simulink model "SF031A_CurrReasbnDiagc"  (R2013b)
settings: Solver=FixedStepDiscrete  SolverMode=SingleTasking  StartTime=0.0  StopTime=1  FixedStep=0.000125  RelTol=1e-3
values from neighbouring files (symbols this model uses):
  ARCHGLBPRM_2MILLISEC_SEC_F32 = DataDict.Constant    [SF031A_CurrReasbnDiagc_DataDict.m]
  ARCHGLBPRM_2PI_ULS_F32 = DataDict.Constant    [SF031A_CurrReasbnDiagc_DataDict.m]
  CurrReasbnDiagcCurrDiagcMotEnvlpTblMax = DataDict.Calibration    [SF031A_CurrReasbnDiagc_DataDict.m]
  CurrReasbnDiagcCurrDiagcPrimErrThd = DataDict.Calibration    [SF031A_CurrReasbnDiagc_DataDict.m]
  CurrReasbnDiagcCurrDiagcSecdryErrThd = DataDict.Calibration    [SF031A_CurrReasbnDiagc_DataDict.m]
  CurrReasbnDiagcCurrDiagcSecdryTqLimThd = DataDict.Calibration    [SF031A_CurrReasbnDiagc_DataDict.m]
  CurrReasbnDiagcDiagFildLim = DataDict.Calibration    [SF031A_CurrReasbnDiagc_DataDict.m]
  CurrReasbnDiagcDiagVltgLpFilEna = DataDict.Calibration    [SF031A_CurrReasbnDiagc_DataDict.m]
  CurrReasbnDiagcLpFilSca = DataDict.Calibration    [SF031A_CurrReasbnDiagc_DataDict.m]
  CurrReasbnDiagcMotVelHiLim = DataDict.Calibration    [SF031A_CurrReasbnDiagc_DataDict.m]
  CurrReasbnDiagcMotVelLoLim = DataDict.Calibration    [SF031A_CurrReasbnDiagc_DataDict.m]
  CurrReasbnDiagcMotVltgQaxDaxFilEna = DataDict.Calibration    [SF031A_CurrReasbnDiagc_DataDict.m]
  CurrReasbnDiagcVelLpFilEna = DataDict.Calibration    [SF031A_CurrReasbnDiagc_DataDict.m]
  ELECGLBPRM_PWMPERDNOMX2_SEC_F32 = DataDict.ConfigParam    [SF031A_CurrReasbnDiagc_DataDict.m]
  NODEBSTEP_CNT_U16 = DataDict.Constant    [SF031A_CurrReasbnDiagc_DataDict.m]
  OffsErrExcdd = DataDict.NTC    [SF031A_CurrReasbnDiagc_DataDict.m]
  ONE_ULS_F32 = DataDict.Constant    [SF031A_CurrReasbnDiagc_DataDict.m]
  ONEOVERTWO_ULS_F32 = DataDict.Constant    [SF031A_CurrReasbnDiagc_DataDict.m]
  SysGlbPrmMotPoleCnt = DataDict.ImprtdCal    [SF031A_CurrReasbnDiagc_DataDict.m]
  TWO_ULS_F32 = DataDict.Constant    [SF031A_CurrReasbnDiagc_DataDict.m]
undefined symbols (not defined in the file or in its folder): NtcSts1
libraries: Fil x8, simulink x6, NxtrLim x3, NxtrMath x2, NexteerUtilities x1
(part 2 of 2)

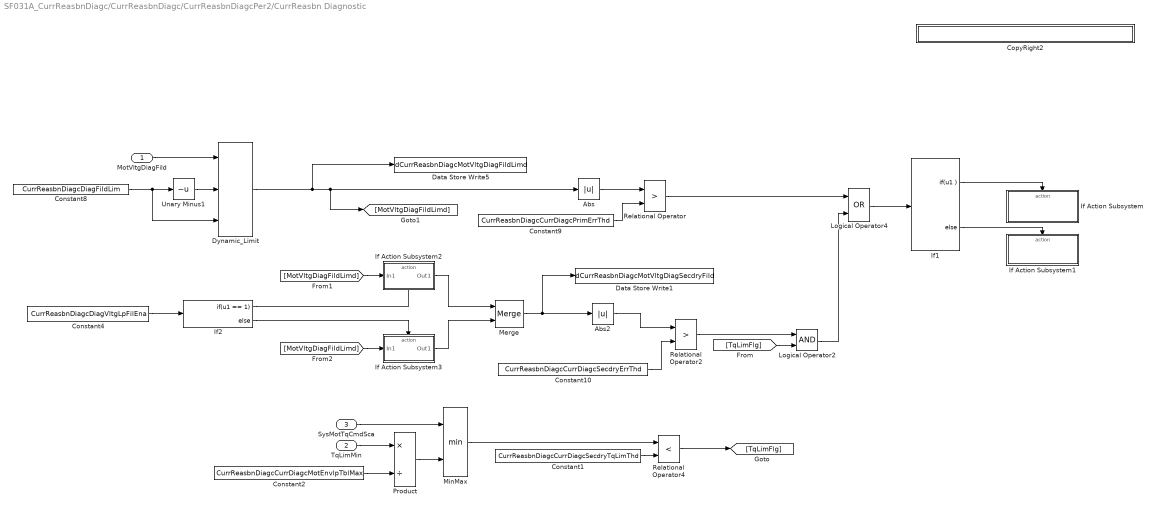
== system SF031A_CurrReasbnDiagc/CurrReasbnDiagc/CurrReasbnDiagcPer2/CurrReasbn Diagnostic ==
  MotVltgDiagFild : Inport
  TqLimMin : Inport  Port=2
  SysMotTqCmdSca : Inport  Port=3
  Abs : Abs
  Abs2 : Abs
  Constant1 : Constant  RequirementInfo="{'linktype_rmi_doors' '0000a538 (/E-STEER Core/SubSystem Specifications/Application Functions/SF031A Current Reasonableness Diagnostic)' '#SF031A_174' 'true' 'REQ:  SF031A_174' '' ; 'linktype_rmi_doors' '0000a538 (/E-STEER Core/SubSystem Specifications/Application Functions/SF031A Current Reasonableness Diagnostic)' '#SF031A_175' 'true' 'REQ:  SF031A_175' '' ; 'linktype_rmi_doors' '0000a538 (/E-STEER Core/SubSystem Specifications/Application Functions/SF031A Current Reasonableness Diagnostic)' '#SF031A_176' 'true' 'REQ:  SF031A_176' '' } %GIDa_b2a65810_aa3d_4d03_8aef_a46f98d57cc6"  Value=CurrReasbnDiagcCurrDiagcSecdryTqLimThd
  Constant10 : Constant  RequirementInfo="{'linktype_rmi_doors' '0000a538 (/E-STEER Core/SubSystem Specifications/Application Functions/SF031A Current Reasonableness Diagnostic)' '#SF031A_59' 'true' 'REQ:  SF031A_59' '' ; 'linktype_rmi_doors' '0000a538 (/E-STEER Core/SubSystem Specifications/Application Functions/SF031A Current Reasonableness Diagnostic)' '#SF031A_169' 'true' 'REQ:  SF031A_169' '' ; 'linktype_rmi_doors' '0000a538 (/E-STEER Core/SubSystem Specifications/Application Functions/SF031A Current Reasonableness Diagnostic)' '#SF031A_170' 'true' 'REQ:  SF031A_170' '' } %GIDa_dec5d4dd_3d51_41a2_8130_bd466e354e12"  Value=CurrReasbnDiagcCurrDiagcSecdryErrThd
  Constant2 : Constant  RequirementInfo="{'linktype_rmi_doors' '0000a538 (/E-STEER Core/SubSystem Specifications/Application Functions/SF031A Current Reasonableness Diagnostic)' '#SF031A_64' 'true' 'REQ:  SF031A_64' '' ; 'linktype_rmi_doors' '0000a538 (/E-STEER Core/SubSystem Specifications/Application Functions/SF031A Current Reasonableness Diagnostic)' '#SF031A_70' 'true' 'REQ:  SF031A_70' '' ; 'linktype_rmi_doors' '0000a538 (/E-STEER Core/SubSystem Specifications/Application Functions/SF031A Current Reasonableness Diagnostic)' '#SF031A_71' 'true' 'REQ:  SF031A_71' '' } %GIDa_c7076ce3_36b3_4c4e_880d_fe3d4c8f6264"  Value=CurrReasbnDiagcCurrDiagcMotEnvlpTblMax
  Constant4 : Constant  RequirementInfo="{'linktype_rmi_doors' '0000a538 (/E-STEER Core/SubSystem Specifications/Application Functions/SF031A Current Reasonableness Diagnostic)' '#SF031A_163' 'true' 'REQ:  SF031A_163' '' ; 'linktype_rmi_doors' '0000a538 (/E-STEER Core/SubSystem Specifications/Application Functions/SF031A Current Reasonableness Diagnostic)' '#SF031A_165' 'true' 'REQ:  SF031A_165' '' ; 'linktype_rmi_doors' '0000a538 (/E-STEER Core/SubSystem Specifications/Application Functions/SF031A Current Reasonableness Diagnostic)' '#SF031A_166' 'true' 'REQ:  SF031A_166' '' } %GIDa_98af6c90_a7cf_453c_acc6_5a96447eaaa3"  Value=CurrReasbnDiagcDiagVltgLpFilEna
  Constant8 : Constant  RequirementInfo="{'linktype_rmi_doors' '0000a538 (/E-STEER Core/SubSystem Specifications/Application Functions/SF031A Current Reasonableness Diagnostic)' '#SF031A_50' 'true' 'REQ:  SF031A_50' '' ; 'linktype_rmi_doors' '0000a538 (/E-STEER Core/SubSystem Specifications/Application Functions/SF031A Current Reasonableness Diagnostic)' '#SF031A_66' 'true' 'REQ:  SF031A_66' '' ; 'linktype_rmi_doors' '0000a538 (/E-STEER Core/SubSystem Specifications/Application Functions/SF031A Current Reasonableness Diagnostic)' '#SF031A_67' 'true' 'REQ:  SF031A_67' '' } %GIDa_7b2e0a81_982f_45cf_af96_5edb94ccb14c"  Value=CurrReasbnDiagcDiagFildLim
  Constant9 : Constant  RequirementInfo="{'linktype_rmi_doors' '0000a538 (/E-STEER Core/SubSystem Specifications/Application Functions/SF031A Current Reasonableness Diagnostic)' '#SF031A_59' 'true' 'REQ:  SF031A_59' '' ; 'linktype_rmi_doors' '0000a538 (/E-STEER Core/SubSystem Specifications/Application Functions/SF031A Current Reasonableness Diagnostic)' '#SF031A_75' 'true' 'REQ:  SF031A_75' '' ; 'linktype_rmi_doors' '0000a538 (/E-STEER Core/SubSystem Specifications/Application Functions/SF031A Current Reasonableness Diagnostic)' '#SF031A_76' 'true' 'REQ:  SF031A_76' '' } %GIDa_fc5a5a33_0937_46a8_b41c_c359f5b2a78c"  Value=CurrReasbnDiagcCurrDiagcPrimErrThd
  CopyRight2 : Subsystem  Description=|  mask(Copyright Information){none=on}
      | Copyright info block.                                               
      |                                                                     
      | Place copyright information at the top of every subsystem in design.
      mask prompts: none "No parameters"
      mask help: Place copyright information at the top of every subsystem in design.
      mask Display:
      | NxtrConf = 'Nexteer Confidential';
      | 
      | sys = bdroot; %handle for the current model ("system")
      | first = get_param(sys,'Created');
      | if(isempty(first))
      |     first = datestr(now,'yyyy');
      | else
      |     first = first(end-3:end);  %year is last four digits
      | end
      | 
      | last = get_param(sys,'LastModifiedDate');
      | if isempty(last)
      |     last = datestr(now,'yyyy');
      | else
      |     last = last(end-3:end);
      | end
      | 
      | if strcmp(first,last)
      |     fprintf('%s -- Copyright %s Nexteer',NxtrConf,first)
      | else
      |     fprintf('%s -- %s%s- %s Nexteer',NxtrConf,char(169),first,last)
      | end
  Data Store Write1 : DataStoreWrite  DataStoreName=dCurrReasbnDiagcMotVltgDiagSecdryFild
  Data Store Write5 : DataStoreWrite  DataStoreName=dCurrReasbnDiagcMotVltgDiagFildLimd
  Dynamic_Limit : NexteerUtilities/Dynamic_Limit  RequirementInfo="{'linktype_rmi_doors' '0000a538 (/E-STEER Core/SubSystem Specifications/Application Functions/SF031A Current Reasonableness Diagnostic)' '#SF031A_51' 'true' 'REQ:  SF031A_51' '' } %GIDa_c9715699_4cf1_4c0d_bb97_eb9e746134b4"
  If Action Subsystem : Subsystem  RequirementInfo="{'linktype_rmi_doors' '0000a538 (/E-STEER Core/SubSystem Specifications/Application Functions/SF031A Current Reasonableness Diagnostic)' '#SF031A_79' 'true' 'REQ:  SF031A_79' '' ; 'linktype_rmi_doors' '0000a538 (/E-STEER Core/SubSystem Specifications/Application Functions/SF031A Current Reasonableness Diagnostic)' '#SF031A_99' 'true' 'REQ:  SF031A_99' '' } %GIDa_5f6b3134_aad8_4144_931a_a09b888c0d15"  TreatAsAtomicUnit=on
  If Action Subsystem1 : Subsystem  RequirementInfo="{'linktype_rmi_doors' '0000a538 (/E-STEER Core/SubSystem Specifications/Application Functions/SF031A Current Reasonableness Diagnostic)' '#SF031A_79' 'true' 'REQ:  SF031A_79' '' ; 'linktype_rmi_doors' '0000a538 (/E-STEER Core/SubSystem Specifications/Application Functions/SF031A Current Reasonableness Diagnostic)' '#SF031A_99' 'true' 'REQ:  SF031A_99' '' } %GIDa_c4fec9d1_35cd_4b3e_8258_ff2c31b4c4bb"  TreatAsAtomicUnit=on
  If Action Subsystem2 : Subsystem  RequirementInfo="{'linktype_rmi_doors' '0000a538 (/E-STEER Core/SubSystem Specifications/Application Functions/SF031A Current Reasonableness Diagnostic)' '#SF031A_164' 'true' 'REQ:  SF031A_164' '' } %GIDa_650c3366_39d1_4640_86a5_1714e62bbfaa"  TreatAsAtomicUnit=on
  If Action Subsystem3 : Subsystem  RequirementInfo="{'linktype_rmi_doors' '0000a538 (/E-STEER Core/SubSystem Specifications/Application Functions/SF031A Current Reasonableness Diagnostic)' '#SF031A_164' 'true' 'REQ:  SF031A_164' '' ; 'linktype_rmi_doors' '0000a538 (/E-STEER Core/SubSystem Specifications/Application Functions/SF031A Current Reasonableness Diagnostic)' '#SF031A_173' 'true' 'REQ:  SF031A_173' '' } %GIDa_947f68a4_3a88_413e_ba90_06cb2007347a"  TreatAsAtomicUnit=on
  If1 : If  RequirementInfo="{'linktype_rmi_doors' '0000a538 (/E-STEER Core/SubSystem Specifications/Application Functions/SF031A Current Reasonableness Diagnostic)' '#SF031A_79' 'true' 'REQ:  SF031A_79' '' ; 'linktype_rmi_doors' '0000a538 (/E-STEER Core/SubSystem Specifications/Application Functions/SF031A Current Reasonableness Diagnostic)' '#SF031A_99' 'true' 'REQ:  SF031A_99' '' } %GIDa_5a3c5e21_bced_48b6_8708_adf8657b0aae"  IfExpression=u1
  If2 : If  RequirementInfo={} %GIDa_1ce7960d_5f42_45cc_8fe4_e04d91b43bbe  IfExpression=u1 == 1
  Logical Operator2 : Logic  RequirementInfo="{'linktype_rmi_doors' '0000a538 (/E-STEER Core/SubSystem Specifications/Application Functions/SF031A Current Reasonableness Diagnostic)' '#SF031A_63' 'true' 'REQ:  SF031A_63' '' } %GIDa_6a4bfa59_21a9_4e81_a797_d4cf70a41219"  AllPortsSameDT=off  OutDataTypeStr=boolean
  Logical Operator4 : Logic  Operator=OR  AllPortsSameDT=off  OutDataTypeStr=boolean
  Merge : Merge  RequirementInfo="{'linktype_rmi_doors' '0000a538 (/E-STEER Core/SubSystem Specifications/Application Functions/SF031A Current Reasonableness Diagnostic)' '#SF031A_164' 'true' 'REQ:  SF031A_164' '' } %GIDa_230e9912_ead3_4162_8555_8f99159292b1"
  MinMax : MinMax  Inputs=2
  Product : Product  Inputs=*/  RndMeth=Zero
  Relational Operator : RelationalOperator  RequirementInfo="{'linktype_rmi_doors' '0000a538 (/E-STEER Core/SubSystem Specifications/Application Functions/SF031A Current Reasonableness Diagnostic)' '#SF031A_58' 'true' 'REQ:  SF031A_58' '' } %GIDa_b53457bd_ac3e_414f_878c_f3118bd509cd"  Operator=>  OutDataTypeStr=boolean
  Relational Operator2 : RelationalOperator  Operator=>  OutDataTypeStr=boolean
  Relational Operator4 : RelationalOperator  Operator=<  OutDataTypeStr=boolean
  Unary Minus1 : UnaryMinus  RequirementInfo={} %GIDa_5127339b_a58c_40c4_bc8f_0902f867244c
  wires:
  MotVltgDiagFild/1 -> Dynamic_Limit/1
  Abs/1 -> Relational Operator/1
  Constant9/1 -> Relational Operator/2
  Abs2/1 -> Relational Operator2/1
  Constant10/1 -> Relational Operator2/2
  Relational Operator2/1 -> Logical Operator2/1
  TqLimMin/1 -> Product/1
  Constant2/1 -> Product/2
  SysMotTqCmdSca/1 -> MinMax/1
  Product/1 -> MinMax/2
  MinMax/1 -> Relational Operator4/1
  Constant1/1 -> Relational Operator4/2
  Relational Operator4/1 -> [TqLimFlg]
  [TqLimFlg] -> Logical Operator2/2
  Unary Minus1/1 -> Dynamic_Limit/2
  Constant8/1 -> Dynamic_Limit/3, Unary Minus1/1
  Merge/1 -> Data Store Write1/1, Abs2/1
  Relational Operator/1 -> Logical Operator4/1
  Logical Operator2/1 -> Logical Operator4/2
  Logical Operator4/1 -> If1/1
  If1/1 -> If Action Subsystem/Action
  If1/2 -> If Action Subsystem1/Action
  If Action Subsystem2/1(Out1) -> Merge/1
  If Action Subsystem3/1(Out1) -> Merge/2
  If2/1 -> If Action Subsystem2/Action
  If2/2 -> If Action Subsystem3/Action
  Constant4/1 -> If2/1
  Dynamic_Limit/1 -> Data Store Write5/1, [MotVltgDiagFildLimd], Abs/1
  [MotVltgDiagFildLimd] -> If Action Subsystem2/1(In1)
  [MotVltgDiagFildLimd] -> If Action Subsystem3/1(In1)

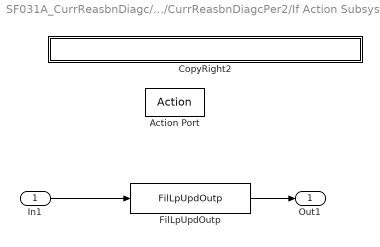
== system SF031A_CurrReasbnDiagc/CurrReasbnDiagc/CurrReasbnDiagcPer2/If Action Subsystem ==
  In1 : Inport
  Action Port : ActionPort  ActionType=then
  CopyRight2 : Subsystem  Description=|  mask(Copyright Information){none=on}
      | Copyright info block.                                               
      |                                                                     
      | Place copyright information at the top of every subsystem in design.
      mask prompts: none "No parameters"
      mask help: Place copyright information at the top of every subsystem in design.
      mask Display:
      | NxtrConf = 'Nexteer Confidential';
      | 
      | sys = bdroot; %handle for the current model ("system")
      | first = get_param(sys,'Created');
      | if(isempty(first))
      |     first = datestr(now,'yyyy');
      | else
      |     first = first(end-3:end);  %year is last four digits
      | end
      | 
      | last = get_param(sys,'LastModifiedDate');
      | if isempty(last)
      |     last = datestr(now,'yyyy');
      | else
      |     last = last(end-3:end);
      | end
      | 
      | if strcmp(first,last)
      |     fprintf('%s -- Copyright %s Nexteer',NxtrConf,first)
      | else
      |     fprintf('%s -- %s%s- %s Nexteer',NxtrConf,char(169),first,last)
      | end
  FilLpUpdOutp : Fil/FilLpUpdOutp  RequirementInfo="{'linktype_rmi_doors' '0000a538 (/E-STEER Core/SubSystem Specifications/Application Functions/SF031A Current Reasonableness Diagnostic)' '#SF031A_139' 'true' 'REQ:  SF031A_139' '' } %GIDa_dc1378f3_074a_4e4d_9443_7b550e8c4f68"  StVar=CurrReasbnMotVelLpFil
      settings: AttributesFormatString=StVar: %<StVar>
  Out1 : Outport
  wires:
  In1/1 -> FilLpUpdOutp/1
  FilLpUpdOutp/1 -> Out1/1

== system SF031A_CurrReasbnDiagc/CurrReasbnDiagc/CurrReasbnDiagcPer2/If Action Subsystem1 ==
  In1 : Inport
  Action Port : ActionPort  ActionType=else
  CopyRight2 : Subsystem  Description=|  mask(Copyright Information){none=on}
      | Copyright info block.                                               
      |                                                                     
      | Place copyright information at the top of every subsystem in design.
      mask prompts: none "No parameters"
      mask help: Place copyright information at the top of every subsystem in design.
      mask Display:
      | NxtrConf = 'Nexteer Confidential';
      | 
      | sys = bdroot; %handle for the current model ("system")
      | first = get_param(sys,'Created');
      | if(isempty(first))
      |     first = datestr(now,'yyyy');
      | else
      |     first = first(end-3:end);  %year is last four digits
      | end
      | 
      | last = get_param(sys,'LastModifiedDate');
      | if isempty(last)
      |     last = datestr(now,'yyyy');
      | else
      |     last = last(end-3:end);
      | end
      | 
      | if strcmp(first,last)
      |     fprintf('%s -- Copyright %s Nexteer',NxtrConf,first)
      | else
      |     fprintf('%s -- %s%s- %s Nexteer',NxtrConf,char(169),first,last)
      | end
  Out1 : Outport
  wires:
  In1/1 -> Out1/1

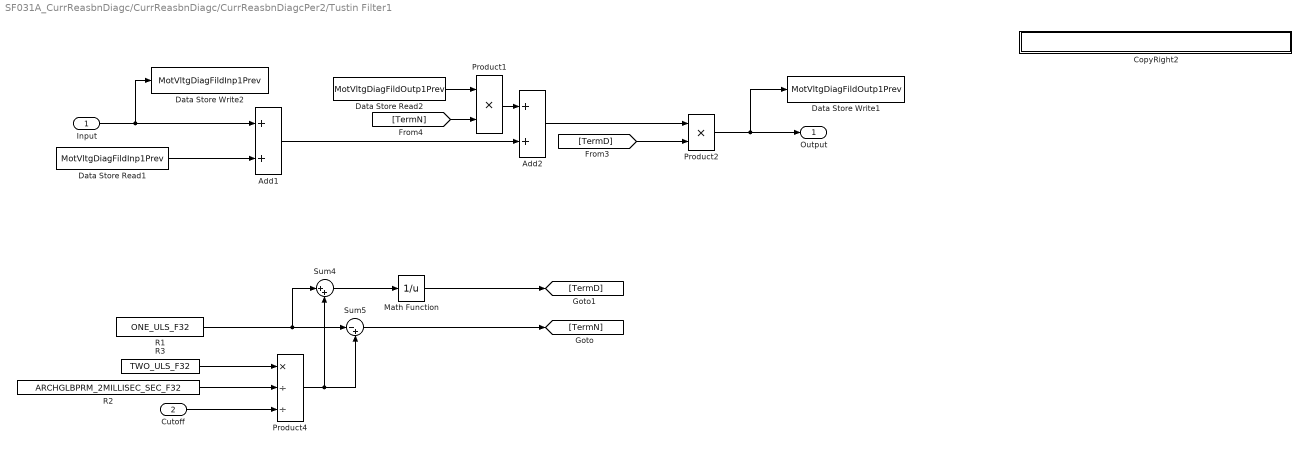
== system SF031A_CurrReasbnDiagc/CurrReasbnDiagc/CurrReasbnDiagcPer2/Tustin Filter1 ==
  Input : Inport
  Cutoff : Inport  Port=2
  Add1 : Sum  RequirementInfo={} %GIDa_c1ed1323_7520_4214_975a_a3195791810c
  Add2 : Sum  RequirementInfo={} %GIDa_391349fe_6344_45b2_b0ed_642c9db5f86a
  CopyRight2 : Subsystem  Description=|  mask(Copyright Information){none=on}
      | Copyright info block.                                               
      |                                                                     
      | Place copyright information at the top of every subsystem in design.
      mask prompts: none "No parameters"
      mask help: Place copyright information at the top of every subsystem in design.
      mask Display:
      | NxtrConf = 'Nexteer Confidential';
      | 
      | sys = bdroot; %handle for the current model ("system")
      | first = get_param(sys,'Created');
      | if(isempty(first))
      |     first = datestr(now,'yyyy');
      | else
      |     first = first(end-3:end);  %year is last four digits
      | end
      | 
      | last = get_param(sys,'LastModifiedDate');
      | if isempty(last)
      |     last = datestr(now,'yyyy');
      | else
      |     last = last(end-3:end);
      | end
      | 
      | if strcmp(first,last)
      |     fprintf('%s -- Copyright %s Nexteer',NxtrConf,first)
      | else
      |     fprintf('%s -- %s%s- %s Nexteer',NxtrConf,char(169),first,last)
      | end
  Data Store Read1 : DataStoreRead  RequirementInfo={} %GIDa_acff8c5f_424e_40b1_98cd_73b420fc5662  Priority=1  DataStoreName=MotVltgDiagFildInp1Prev
      settings: AttributesFormatString=Priority=%<Priority>
  Data Store Read2 : DataStoreRead  RequirementInfo={} %GIDa_5121f4d0_20eb_4589_9d60_13579401b42f  Priority=2  DataStoreName=MotVltgDiagFildOutp1Prev
  Data Store Write1 : DataStoreWrite  RequirementInfo={} %GIDa_db53aa91_fff2_4720_89d2_150c497ea7b0  DataStoreName=MotVltgDiagFildOutp1Prev
  Data Store Write2 : DataStoreWrite  RequirementInfo={} %GIDa_6c53b441_2320_40f4_a5f5_e21fd189c901  Priority=2  DataStoreName=MotVltgDiagFildInp1Prev
  Math Function : Math  Operator=reciprocal  SaturateOnIntegerOverflow=on
  Product1 : Product
  Product2 : Product  Inputs=**
  Product4 : Product  Inputs=*//
  R1 : Constant  Value=ONE_ULS_F32
  R2 : Constant  Value=ARCHGLBPRM_2MILLISEC_SEC_F32
  R3 : Constant  Value=TWO_ULS_F32
  Sum4 : Sum  Inputs=|++
  Sum5 : Sum  Inputs=|-+
  Output : Outport
  wires:
  Add1/1 -> Add2/2
  Input/1 -> Data Store Write2/1, Add1/1
  Add2/1 -> Product2/1
  Data Store Read1/1 -> Add1/2
  [TermD] -> Product2/2
  [TermN] -> Product1/2
  Product1/1 -> Add2/1
  Product2/1 -> Output/1, Data Store Write1/1
  Data Store Read2/1 -> Product1/1
  R3/1 -> Product4/1
  R2/1 -> Product4/2
  Sum5/1 -> [TermN]
  Cutoff/1 -> Product4/3
  Product4/1 -> Sum4/2, Sum5/2
  R1/1 -> Sum4/1, Sum5/1
  Sum4/1 -> Math Function/1
  Math Function/1 -> [TermD]

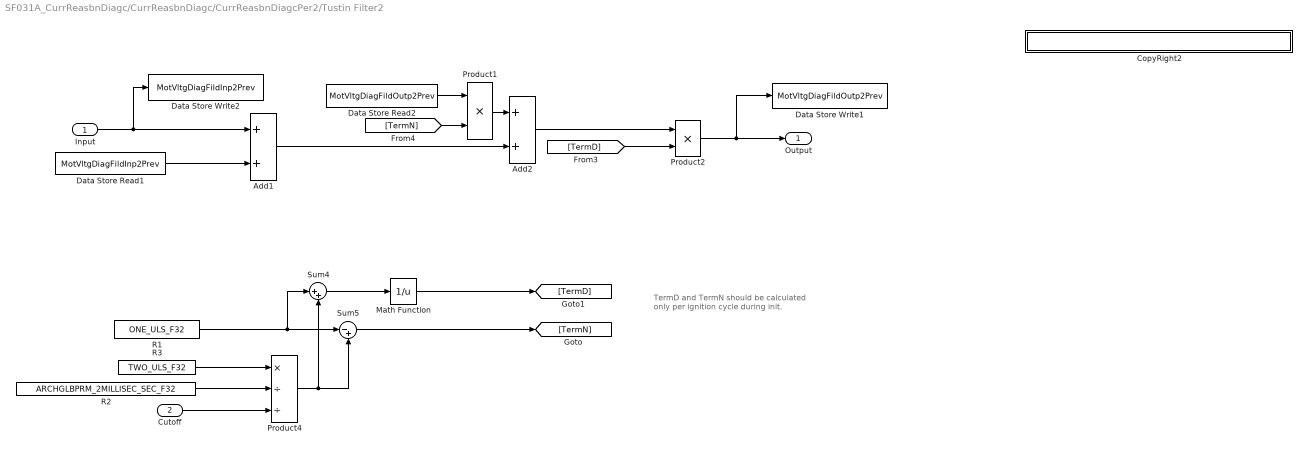
== system SF031A_CurrReasbnDiagc/CurrReasbnDiagc/CurrReasbnDiagcPer2/Tustin Filter2 ==
  note: TermD and TermN should be calculated
      | only per ignition cycle during init.
  Input : Inport
  Cutoff : Inport  Port=2
  Add1 : Sum  RequirementInfo={} %GIDa_a894f2e9_b801_4d1f_9d93_6f4ee7bb8e0e
  Add2 : Sum  RequirementInfo={} %GIDa_f86e10b4_b110_4ce5_a15b_c460bb4a4b0c
  CopyRight2 : Subsystem  Description=|  mask(Copyright Information){none=on}
      | Copyright info block.                                               
      |                                                                     
      | Place copyright information at the top of every subsystem in design.
      mask prompts: none "No parameters"
      mask help: Place copyright information at the top of every subsystem in design.
      mask Display:
      | NxtrConf = 'Nexteer Confidential';
      | 
      | sys = bdroot; %handle for the current model ("system")
      | first = get_param(sys,'Created');
      | if(isempty(first))
      |     first = datestr(now,'yyyy');
      | else
      |     first = first(end-3:end);  %year is last four digits
      | end
      | 
      | last = get_param(sys,'LastModifiedDate');
      | if isempty(last)
      |     last = datestr(now,'yyyy');
      | else
      |     last = last(end-3:end);
      | end
      | 
      | if strcmp(first,last)
      |     fprintf('%s -- Copyright %s Nexteer',NxtrConf,first)
      | else
      |     fprintf('%s -- %s%s- %s Nexteer',NxtrConf,char(169),first,last)
      | end
  Data Store Read1 : DataStoreRead  RequirementInfo={} %GIDa_d021f800_ff34_4acd_b134_b92c72ff1596  Priority=1  DataStoreName=MotVltgDiagFildInp2Prev
      settings: AttributesFormatString=Priority=%<Priority>
  Data Store Read2 : DataStoreRead  RequirementInfo={} %GIDa_f19a8e9b_a536_43d5_a481_789e91f0b73a  DataStoreName=MotVltgDiagFildOutp2Prev
  Data Store Write1 : DataStoreWrite  RequirementInfo={} %GIDa_1d248a82_b691_41c0_a9ec_626bfc5b8f5b  DataStoreName=MotVltgDiagFildOutp2Prev
  Data Store Write2 : DataStoreWrite  RequirementInfo={} %GIDa_f73d3bf2_86df_4e02_87ff_f73e483fc73f  Priority=2  DataStoreName=MotVltgDiagFildInp2Prev
  Math Function : Math  Operator=reciprocal  SaturateOnIntegerOverflow=on
  Product1 : Product
  Product2 : Product  Inputs=**
  Product4 : Product  Inputs=*//
  R1 : Constant  Value=ONE_ULS_F32
  R2 : Constant  Value=ARCHGLBPRM_2MILLISEC_SEC_F32
  R3 : Constant  Value=TWO_ULS_F32
  Sum4 : Sum  Inputs=|++
  Sum5 : Sum  Inputs=|-+
  Output : Outport
  wires:
  Math Function/1 -> [TermD]
  Sum4/1 -> Math Function/1
  R1/1 -> Sum5/1, Sum4/1
  Product4/1 -> Sum5/2, Sum4/2
  Cutoff/1 -> Product4/3
  Sum5/1 -> [TermN]
  R2/1 -> Product4/2
  R3/1 -> Product4/1
  Data Store Read2/1 -> Product1/1
  Product2/1 -> Data Store Write1/1, Output/1
  Product1/1 -> Add2/1
  [TermN] -> Product1/2
  [TermD] -> Product2/2
  Data Store Read1/1 -> Add1/2
  Add2/1 -> Product2/1
  Input/1 -> Add1/1, Data Store Write2/1
  Add1/1 -> Add2/2

== system SF031A_CurrReasbnDiagc/CurrReasbnDiagc/CurrReasbnDiagcPer1/If Action Subsystem/CopyRight2 ==

== system SF031A_CurrReasbnDiagc/CurrReasbnDiagc/CurrReasbnDiagcPer1/If Action Subsystem1/CopyRight2 ==

== system SF031A_CurrReasbnDiagc/CurrReasbnDiagc/CurrReasbnDiagcPer1/If Action Subsystem2/CopyRight2 ==

== system SF031A_CurrReasbnDiagc/CurrReasbnDiagc/CurrReasbnDiagcPer1/If Action Subsystem3/CopyRight2 ==

== system SF031A_CurrReasbnDiagc/CurrReasbnDiagc/CurrReasbnDiagcPer2/CurrReasbn Diagnostic/CopyRight2 ==

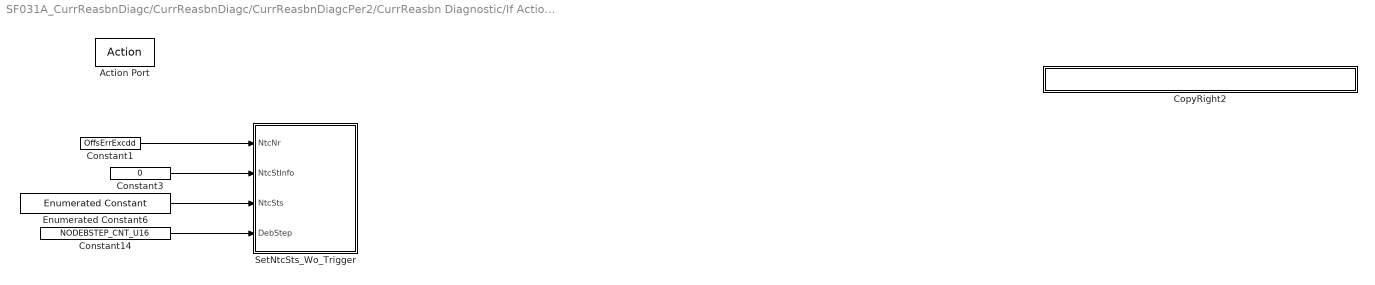
== system SF031A_CurrReasbnDiagc/CurrReasbnDiagc/CurrReasbnDiagcPer2/CurrReasbn Diagnostic/If Action Subsystem ==
  Action Port : ActionPort  ActionType=then
  Constant1 : Constant  RequirementInfo={} %GIDa_5d3a90a6_ef0f_4ce3_bbe2_3a5c51fd87e0  Value=OffsErrExcdd
  Constant14 : Constant  RequirementInfo={} %GIDa_33859d68_b904_4f0e_88b8_20d9e6783e52  Value=NODEBSTEP_CNT_U16
  Constant3 : Constant  RequirementInfo={} %GIDa_47ea69f8_b500_4b37_af00_458de788a20b  Value=0
  CopyRight2 : Subsystem  Description=|  mask(Copyright Information){none=on}
      | Copyright info block.                                               
      |                                                                     
      | Place copyright information at the top of every subsystem in design.
      mask prompts: none "No parameters"
      mask help: Place copyright information at the top of every subsystem in design.
      mask Display:
      | NxtrConf = 'Nexteer Confidential';
      | 
      | sys = bdroot; %handle for the current model ("system")
      | first = get_param(sys,'Created');
      | if(isempty(first))
      |     first = datestr(now,'yyyy');
      | else
      |     first = first(end-3:end);  %year is last four digits
      | end
      | 
      | last = get_param(sys,'LastModifiedDate');
      | if isempty(last)
      |     last = datestr(now,'yyyy');
      | else
      |     last = last(end-3:end);
      | end
      | 
      | if strcmp(first,last)
      |     fprintf('%s -- Copyright %s Nexteer',NxtrConf,first)
      | else
      |     fprintf('%s -- %s%s- %s Nexteer',NxtrConf,char(169),first,last)
      | end
  Enumerated Constant6 : simulink/Sources/Enumerated Constant  RequirementInfo={} %GIDa_64488fd3_fc07_4748_b05f_e60f2142f6b3  OutDataTypeStr=Enum: NtcSts1  Value=NtcSts1.NTCSTS_FAILD  SampleTime=inf
  SetNtcSts_Wo_Trigger : Subsystem  mask(SetNTC_WOT){}
      mask help: SetNTC library block
  wires:
  Constant3/1 -> SetNtcSts_Wo_Trigger/2(NtcStInfo)
  Constant1/1 -> SetNtcSts_Wo_Trigger/1(NtcNr)
  Enumerated Constant6/1 -> SetNtcSts_Wo_Trigger/3(NtcSts)
  Constant14/1 -> SetNtcSts_Wo_Trigger/4(DebStep)

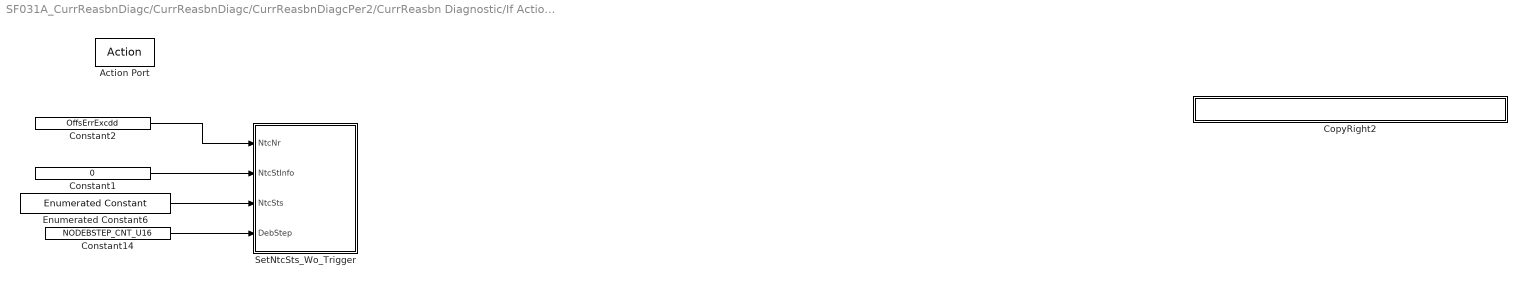
== system SF031A_CurrReasbnDiagc/CurrReasbnDiagc/CurrReasbnDiagcPer2/CurrReasbn Diagnostic/If Action Subsystem1 ==
  Action Port : ActionPort  ActionType=else
  Constant1 : Constant  RequirementInfo={} %GIDa_24eb1b5a_22c7_46ba_adb0_ad7e63d13c99  Value=0
  Constant14 : Constant  RequirementInfo={} %GIDa_5b0baf7c_ba6e_40e7_850d_b7b4fb97f50b  Value=NODEBSTEP_CNT_U16
  Constant2 : Constant  RequirementInfo={} %GIDa_fba0a50e_4599_4a09_9322_fb457d04940d  Value=OffsErrExcdd
  CopyRight2 : Subsystem  Description=|  mask(Copyright Information){none=on}
      | Copyright info block.                                               
      |                                                                     
      | Place copyright information at the top of every subsystem in design.
      mask prompts: none "No parameters"
      mask help: Place copyright information at the top of every subsystem in design.
      mask Display:
      | NxtrConf = 'Nexteer Confidential';
      | 
      | sys = bdroot; %handle for the current model ("system")
      | first = get_param(sys,'Created');
      | if(isempty(first))
      |     first = datestr(now,'yyyy');
      | else
      |     first = first(end-3:end);  %year is last four digits
      | end
      | 
      | last = get_param(sys,'LastModifiedDate');
      | if isempty(last)
      |     last = datestr(now,'yyyy');
      | else
      |     last = last(end-3:end);
      | end
      | 
      | if strcmp(first,last)
      |     fprintf('%s -- Copyright %s Nexteer',NxtrConf,first)
      | else
      |     fprintf('%s -- %s%s- %s Nexteer',NxtrConf,char(169),first,last)
      | end
  Enumerated Constant6 : simulink/Sources/Enumerated Constant  RequirementInfo={} %GIDa_5262f637_bae4_4e55_941b_09db5c0c0008  OutDataTypeStr=Enum: NtcSts1  Value=NtcSts1.NTCSTS_PASSD  SampleTime=inf
  SetNtcSts_Wo_Trigger : Subsystem  mask(SetNTC_WOT){}
      mask help: SetNTC library block
  wires:
  Constant14/1 -> SetNtcSts_Wo_Trigger/4(DebStep)
  Enumerated Constant6/1 -> SetNtcSts_Wo_Trigger/3(NtcSts)
  Constant2/1 -> SetNtcSts_Wo_Trigger/1(NtcNr)
  Constant1/1 -> SetNtcSts_Wo_Trigger/2(NtcStInfo)

== system SF031A_CurrReasbnDiagc/CurrReasbnDiagc/CurrReasbnDiagcPer2/CurrReasbn Diagnostic/If Action Subsystem2 ==
  In1 : Inport
  Action Port : ActionPort  ActionType=then
  CopyRight2 : Subsystem  Description=|  mask(Copyright Information){none=on}
      | Copyright info block.                                               
      |                                                                     
      | Place copyright information at the top of every subsystem in design.
      mask prompts: none "No parameters"
      mask help: Place copyright information at the top of every subsystem in design.
      mask Display:
      | NxtrConf = 'Nexteer Confidential';
      | 
      | sys = bdroot; %handle for the current model ("system")
      | first = get_param(sys,'Created');
      | if(isempty(first))
      |     first = datestr(now,'yyyy');
      | else
      |     first = first(end-3:end);  %year is last four digits
      | end
      | 
      | last = get_param(sys,'LastModifiedDate');
      | if isempty(last)
      |     last = datestr(now,'yyyy');
      | else
      |     last = last(end-3:end);
      | end
      | 
      | if strcmp(first,last)
      |     fprintf('%s -- Copyright %s Nexteer',NxtrConf,first)
      | else
      |     fprintf('%s -- %s%s- %s Nexteer',NxtrConf,char(169),first,last)
      | end
  FilLpUpdOutp : Fil/FilLpUpdOutp  RequirementInfo="{'linktype_rmi_doors' '0000a538 (/E-STEER Core/SubSystem Specifications/Application Functions/SF031A Current Reasonableness Diagnostic)' '#SF031A_167' 'true' 'REQ:  SF031A_167' '' } %GIDa_10f79e64_b568_417a_9eda_1be3b253ee35"  StVar=DiagVltgLpFil
      settings: AttributesFormatString=StVar: %<StVar>
  Out1 : Outport
  wires:
  In1/1 -> FilLpUpdOutp/1
  FilLpUpdOutp/1 -> Out1/1

== system SF031A_CurrReasbnDiagc/CurrReasbnDiagc/CurrReasbnDiagcPer2/CurrReasbn Diagnostic/If Action Subsystem3 ==
  In1 : Inport
  Action Port : ActionPort  ActionType=else
  CopyRight2 : Subsystem  Description=|  mask(Copyright Information){none=on}
      | Copyright info block.                                               
      |                                                                     
      | Place copyright information at the top of every subsystem in design.
      mask prompts: none "No parameters"
      mask help: Place copyright information at the top of every subsystem in design.
      mask Display:
      | NxtrConf = 'Nexteer Confidential';
      | 
      | sys = bdroot; %handle for the current model ("system")
      | first = get_param(sys,'Created');
      | if(isempty(first))
      |     first = datestr(now,'yyyy');
      | else
      |     first = first(end-3:end);  %year is last four digits
      | end
      | 
      | last = get_param(sys,'LastModifiedDate');
      | if isempty(last)
      |     last = datestr(now,'yyyy');
      | else
      |     last = last(end-3:end);
      | end
      | 
      | if strcmp(first,last)
      |     fprintf('%s -- Copyright %s Nexteer',NxtrConf,first)
      | else
      |     fprintf('%s -- %s%s- %s Nexteer',NxtrConf,char(169),first,last)
      | end
  Out1 : Outport
  wires:
  In1/1 -> Out1/1

== system SF031A_CurrReasbnDiagc/CurrReasbnDiagc/CurrReasbnDiagcPer2/If Action Subsystem/CopyRight2 ==

== system SF031A_CurrReasbnDiagc/CurrReasbnDiagc/CurrReasbnDiagcPer2/If Action Subsystem1/CopyRight2 ==

== system SF031A_CurrReasbnDiagc/CurrReasbnDiagc/CurrReasbnDiagcPer2/Tustin Filter1/CopyRight2 ==

== system SF031A_CurrReasbnDiagc/CurrReasbnDiagc/CurrReasbnDiagcPer2/Tustin Filter2/CopyRight2 ==

== system SF031A_CurrReasbnDiagc/CurrReasbnDiagc/CurrReasbnDiagcPer2/CurrReasbn Diagnostic/If Action Subsystem/CopyRight2 ==

== system SF031A_CurrReasbnDiagc/CurrReasbnDiagc/CurrReasbnDiagcPer2/CurrReasbn Diagnostic/If Action Subsystem/SetNtcSts_Wo_Trigger ==
  NtcNr : Inport
  NtcStInfo : Inport  Port=2
  NtcSts : Inport  Port=3
  DebStep : Inport  Port=4
  SetNtcSts : Subsystem  RequirementInfo={} %GIDa_c862e468_89c6_4515_bb27_39c0b9395d5b  TreatAsAtomicUnit=on
      settings: RTWSystemCode=Inline
  wires:
  NtcStInfo/1 -> SetNtcSts/2(NtcStInfo)
  DebStep/1 -> SetNtcSts/4(DebStep)
  NtcSts/1 -> SetNtcSts/3(NtcSts)
  NtcNr/1 -> SetNtcSts/1(NtcNr)  "NtcNr"

== system SF031A_CurrReasbnDiagc/CurrReasbnDiagc/CurrReasbnDiagcPer2/CurrReasbn Diagnostic/If Action Subsystem1/CopyRight2 ==

== system SF031A_CurrReasbnDiagc/CurrReasbnDiagc/CurrReasbnDiagcPer2/CurrReasbn Diagnostic/If Action Subsystem1/SetNtcSts_Wo_Trigger ==
  NtcNr : Inport
  NtcStInfo : Inport  Port=2
  NtcSts : Inport  Port=3
  DebStep : Inport  Port=4
  SetNtcSts : Subsystem  RequirementInfo={} %GIDa_f812c850_00c8_47c1_8947_bf76584e5060  TreatAsAtomicUnit=on
      settings: RTWSystemCode=Inline
  wires:
  NtcNr/1 -> SetNtcSts/1(NtcNr)  "NtcNr"
  NtcSts/1 -> SetNtcSts/3(NtcSts)
  DebStep/1 -> SetNtcSts/4(DebStep)
  NtcStInfo/1 -> SetNtcSts/2(NtcStInfo)

== system SF031A_CurrReasbnDiagc/CurrReasbnDiagc/CurrReasbnDiagcPer2/CurrReasbn Diagnostic/If Action Subsystem2/CopyRight2 ==

== system SF031A_CurrReasbnDiagc/CurrReasbnDiagc/CurrReasbnDiagcPer2/CurrReasbn Diagnostic/If Action Subsystem3/CopyRight2 ==

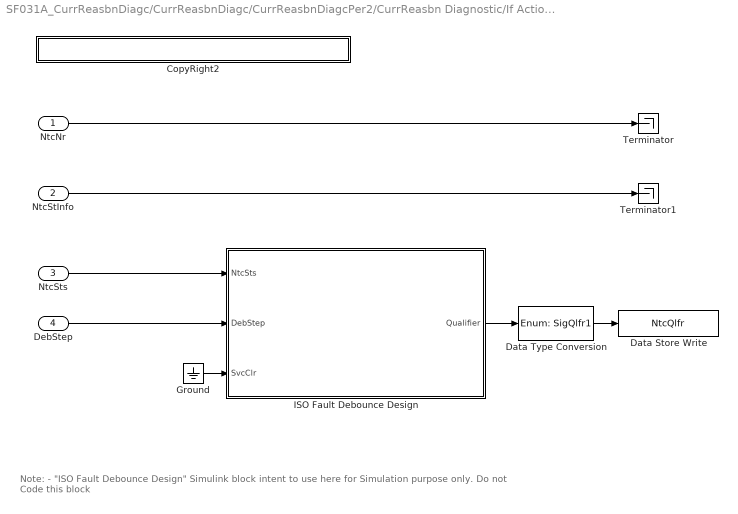
== system SF031A_CurrReasbnDiagc/CurrReasbnDiagc/CurrReasbnDiagcPer2/CurrReasbn Diagnostic/If Action Subsystem/SetNtcSts_Wo_Trigger/SetNtcSts ==
  note: Note:
      |
      | - "ISO Fault Debounce Design" Simulink block intent to use here for Simulation purpose only. Do not Code this block
  NtcNr : Inport
  NtcStInfo : Inport  Port=2
  NtcSts : Inport  Port=3
  DebStep : Inport  Port=4
  CopyRight2 : Subsystem  Description=|  mask(Copyright Information){none=on}
      | Copyright info block.                                               
      |                                                                     
      | Place copyright information at the top of every subsystem in design.
      mask prompts: none "No parameters"
      mask help: Place copyright information at the top of every subsystem in design.
      mask Display:
      | NxtrConf = 'Nexteer Confidential';
      | 
      | sys = bdroot; %handle for the current model ("system")
      | first = get_param(sys,'Created');
      | first = first(end-3:end);  %year is last four digits
      | 
      | last = get_param(sys,'LastModifiedDate');
      | if isempty(last)
      |     last = datestr(now,'yyyy');
      | else
      |     last = last(end-3:end);
      | end
      | 
      | if strcmp(first,last)
      |     fprintf('%s -- Copyright %s Nexteer',NxtrConf,first)
      | else
      |     fprintf('%s -- %s%s- %s Nexteer',NxtrConf,char(169),first,last)
      | end
  Data Store Write : DataStoreWrite  DataStoreName=NtcQlfr
  Data Type Conversion : DataTypeConversion  OutDataTypeStr=Enum: SigQlfr1
  Ground : Ground
  ISO Fault Debounce Design : Stateflow chart  TreatAsAtomicUnit=on
      settings: AttributesFormatString=|
      | Simulation Purpose Only.
      | Do Not Code this block
      | Diagnostic Manager Owns this requirement
  Terminator : Terminator
  Terminator1 : Terminator
  wires:
  Ground/1 -> ISO Fault Debounce Design/3(SvcClr)
  ISO Fault Debounce Design/1(Qualifier) -> Data Type Conversion/1
  DebStep/1 -> ISO Fault Debounce Design/2(DebStep)
  NtcSts/1 -> ISO Fault Debounce Design/1(NtcSts)
  NtcNr/1 -> Terminator/1
  NtcStInfo/1 -> Terminator1/1
  Data Type Conversion/1 -> Data Store Write/1

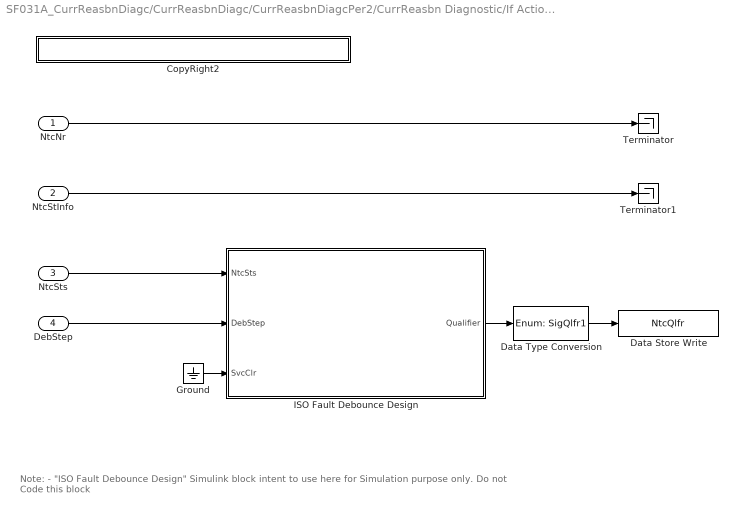
== system SF031A_CurrReasbnDiagc/CurrReasbnDiagc/CurrReasbnDiagcPer2/CurrReasbn Diagnostic/If Action Subsystem1/SetNtcSts_Wo_Trigger/SetNtcSts ==
  note: Note:
      |
      | - "ISO Fault Debounce Design" Simulink block intent to use here for Simulation purpose only. Do not Code this block
  NtcNr : Inport
  NtcStInfo : Inport  Port=2
  NtcSts : Inport  Port=3
  DebStep : Inport  Port=4
  CopyRight2 : Subsystem  Description=|  mask(Copyright Information){none=on}
      | Copyright info block.                                               
      |                                                                     
      | Place copyright information at the top of every subsystem in design.
      mask prompts: none "No parameters"
      mask help: Place copyright information at the top of every subsystem in design.
      mask Display:
      | NxtrConf = 'Nexteer Confidential';
      | 
      | sys = bdroot; %handle for the current model ("system")
      | first = get_param(sys,'Created');
      | first = first(end-3:end);  %year is last four digits
      | 
      | last = get_param(sys,'LastModifiedDate');
      | if isempty(last)
      |     last = datestr(now,'yyyy');
      | else
      |     last = last(end-3:end);
      | end
      | 
      | if strcmp(first,last)
      |     fprintf('%s -- Copyright %s Nexteer',NxtrConf,first)
      | else
      |     fprintf('%s -- %s%s- %s Nexteer',NxtrConf,char(169),first,last)
      | end
  Data Store Write : DataStoreWrite  DataStoreName=NtcQlfr
  Data Type Conversion : DataTypeConversion  OutDataTypeStr=Enum: SigQlfr1
  Ground : Ground
  ISO Fault Debounce Design : Stateflow chart  TreatAsAtomicUnit=on
      settings: AttributesFormatString=|
      | Simulation Purpose Only.
      | Do Not Code this block
      | Diagnostic Manager Owns this requirement
  Terminator : Terminator
  Terminator1 : Terminator
  wires:
  NtcStInfo/1 -> Terminator1/1
  NtcNr/1 -> Terminator/1
  NtcSts/1 -> ISO Fault Debounce Design/1(NtcSts)
  DebStep/1 -> ISO Fault Debounce Design/2(DebStep)
  ISO Fault Debounce Design/1(Qualifier) -> Data Type Conversion/1
  Ground/1 -> ISO Fault Debounce Design/3(SvcClr)
  Data Type Conversion/1 -> Data Store Write/1

== system SF031A_CurrReasbnDiagc/CurrReasbnDiagc/CurrReasbnDiagcPer2/CurrReasbn Diagnostic/If Action Subsystem/SetNtcSts_Wo_Trigger/SetNtcSts/CopyRight2 ==

== system SF031A_CurrReasbnDiagc/CurrReasbnDiagc/CurrReasbnDiagcPer2/CurrReasbn Diagnostic/If Action Subsystem1/SetNtcSts_Wo_Trigger/SetNtcSts/CopyRight2 ==

== stateflow chart SF031A_CurrReasbnDiagc/CurrReasbnDiagc/CurrReasbnDiagcPer2/CurrReasbn Diagnostic/If Action Subsystem/SetNtcSts_Wo_Trigger/SetNtcSts/ISO Fault Debounce Design ==
  note: NTCSTS_PASSD           (0)
      | NTCSTS_FAILD             (1)
      | NTCSTS_PREPASSD   (2)
      | NTCSTS_PREFAILD     (3)
      |
      | SIGQLFR_NORES        (0)
      | SIGQLFR_PASSD         (1)
      | SIGQLFR_FAILD           (2)
  note: Pass Loop
  note: Fail Loop
  note: 
  (default) -> (junction 89)
  (junction 89) -> (junction 95) [order 1] : [NtcSts ==3]
  (junction 89) -> (junction 93) [order 2] : [NtcSts ==2]
  (junction 89) -> (junction 141) [order 3] : [NtcSts ==1]
      | { ErrAcc = 32767;
      | Qualifier =2;
      |  }
  (junction 89) -> (junction 141) [order 4] : [NtcSts ==0]
      | { ErrAcc = -32768;
      | Qualifier=1;
      | }
  (junction 95) -> (junction 103) [order 2]
  (junction 95) -> (junction 111) [order 1] : [ErrAcc <=0]
      | {ErrAcc = DebStep;}
  (junction 93) -> (junction 123) [order 2] : {
      | ErrAcc = ErrAcc - DebStep;
      | }
  (junction 93) -> (junction 123) [order 1] : [(ErrAcc - DebStep) <= -32768]
      | { ErrAcc = -32768;
      | Qualifier=1;
      | }
  (junction 103) -> (junction 111) [order 1] : [(ErrAcc + DebStep) <32767]
      | {ErrAcc = ErrAcc + DebStep;}
  (junction 103) -> (junction 111) [order 2] : {ErrAcc = 32767;
      | Qualifier =2;}
  (junction 123) -> (junction 141)
  (junction 111) -> (junction 141)
  (junction 141) -> (junction 159) [order 2] : {ErrAcc = 0;
      | Qualifier =0;
      | }
  (junction 141) -> (junction 159) [order 1] : [SvcClr ==0]
  data: NtcSts input Enum: NtcSts1; Qualifier output uint8; DebStep input uint16; ErrAcc local single; SvcClr input

== stateflow chart SF031A_CurrReasbnDiagc/CurrReasbnDiagc/CurrReasbnDiagcPer2/CurrReasbn Diagnostic/If Action Subsystem1/SetNtcSts_Wo_Trigger/SetNtcSts/ISO Fault Debounce Design ==
  note: NTCSTS_PASSD           (0)
      | NTCSTS_FAILD             (1)
      | NTCSTS_PREPASSD   (2)
      | NTCSTS_PREFAILD     (3)
      |
      | SIGQLFR_NORES        (0)
      | SIGQLFR_PASSD         (1)
      | SIGQLFR_FAILD           (2)
  note: Pass Loop
  note: Fail Loop
  note: 
  (default) -> (junction 89)
  (junction 89) -> (junction 95) [order 1] : [NtcSts ==3]
  (junction 89) -> (junction 93) [order 2] : [NtcSts ==2]
  (junction 89) -> (junction 141) [order 3] : [NtcSts ==1]
      | { ErrAcc = 32767;
      | Qualifier =2;
      |  }
  (junction 89) -> (junction 141) [order 4] : [NtcSts ==0]
      | { ErrAcc = -32768;
      | Qualifier=1;
      | }
  (junction 95) -> (junction 103) [order 2]
  (junction 95) -> (junction 111) [order 1] : [ErrAcc <=0]
      | {ErrAcc = DebStep;}
  (junction 93) -> (junction 123) [order 2] : {
      | ErrAcc = ErrAcc - DebStep;
      | }
  (junction 93) -> (junction 123) [order 1] : [(ErrAcc - DebStep) <= -32768]
      | { ErrAcc = -32768;
      | Qualifier=1;
      | }
  (junction 103) -> (junction 111) [order 1] : [(ErrAcc + DebStep) <32767]
      | {ErrAcc = ErrAcc + DebStep;}
  (junction 103) -> (junction 111) [order 2] : {ErrAcc = 32767;
      | Qualifier =2;}
  (junction 123) -> (junction 141)
  (junction 111) -> (junction 141)
  (junction 141) -> (junction 159) [order 2] : {ErrAcc = 0;
      | Qualifier =0;
      | }
  (junction 141) -> (junction 159) [order 1] : [SvcClr ==0]
  data: NtcSts input Enum: NtcSts1; Qualifier output uint8; DebStep input uint16; ErrAcc local single; SvcClr input
